simulink model "mg337440"  (Simulink 6.6)
settings: Solver=ode45  StartTime=0.0  StopTime=10.0  RelTol=1e-3
model workspace (MAT data in the model file):
  test : struct (value not decoded)
settings Model: Creator=sethp  LastModifiedBy=mshakeri  ExtModeAutoUpdateStatusClock=off
settings OptimizationCC: InlineParams=on
settings DebuggingCC: MultiTaskDSMMsg=warning  MultiTaskCondExecSysMsg=none  StrictBusMsg=ErrorLevel1
settings RTWCC: IncludeERTFirstTime=on

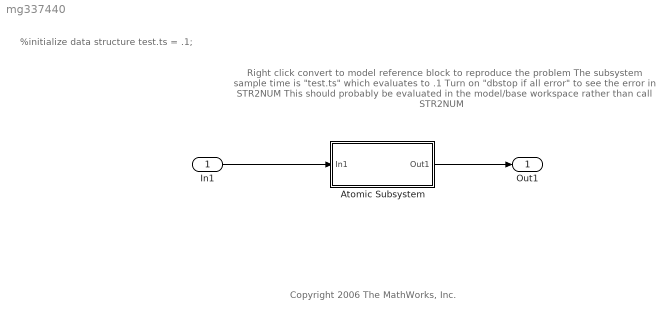
== system mg337440 ==
  note: %initialize data structure
      | test.ts = .1;
  note: Right click convert to model reference block to reproduce the problem
      | The subsystem sample time is "test.ts" which evaluates to .1
      | Turn on "dbstop if all error" to see the error in STR2NUM
      | This should probably be evaluated in the model/base workspace rather than call STR2NUM
  note: Copyright 2006 The MathWorks, Inc.
  In1 : Inport
  Atomic Subsystem : Subsystem  TreatAsAtomicUnit=on  SystemSampleTime=test.ts
  Out1 : Outport
  wires:
  In1/1 -> Atomic Subsystem/1(In1)
  Atomic Subsystem/1(Out1) -> Out1/1

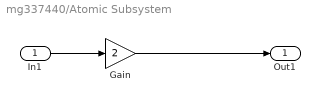
== system mg337440/Atomic Subsystem ==
  In1 : Inport
  Gain : Gain  Gain=2
  Out1 : Outport
  wires:
  In1/1 -> Gain/1
  Gain/1 -> Out1/1
